simulink model "PartA_19EE10039"  (R2021a)
settings: Solver=FixedStepAuto  StartTime=0.0  StopTime=0.08  FixedStep=1e-7  MaxStep=1e-7  RelTol=1e-6
libraries: simulink x6, spsMonostableLib x6, spsVoltageMeasurementLib x3, spsThreePhaseSourceLib x1, spsThreePhaseTransformerTwoWindingsLib x1, spspowerguiLib x1
settings Model: Creator=Triptendu  LastModifiedBy=mansi
settings SolverCC: AlgebraicLoopSolver=TrustRegion
settings DataIOCC: ReturnWorkspaceOutputs=off
settings DebuggingCC: SFMachineParentedDataDiag=warning

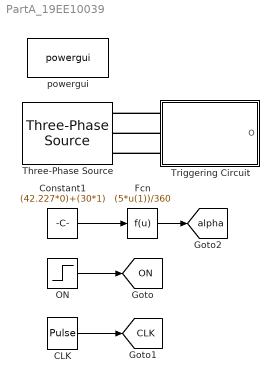
== system PartA_19EE10039 ==
  CLK : DiscretePulseGenerator  PulseType=Time based  Period=40e-6  PulseWidth=50
  Constant1 : Constant  Value=(42.227*0)+(30*1)
  Fcn : Fcn  Expr=(5*u(1))/360
  ON : Step  Time=0.02  SampleTime=0
  Three-Phase Source : spsThreePhaseSourceLib/Three-Phase Source  InternalConnection=Y  VoltagePhases=off  Voltage=220  PhaseAngle=0  Voltage_phases=[25e3 25e3 25e3]/sqrt(3)  PhaseAngles_phases=[0 -120 +120]  Frequency=50  NonIdealSource=on  SpecifyImpedance=off  Resistance=0  Inductance=0  ShortCircuitLevel=100e6  BaseVoltage=220  XRratio=7  BusType=swing  Pref=10e3  Qref=0  Prefabc=[10e3, 10e3, 10e3]  Qrefabc=[0, 0, 0]  Qmin=-inf  Qmax=inf
  Triggering Circuit : Subsystem
  powergui : spspowerguiLib/powergui  Priority=1  SimulationMode=Discrete  SampleTime=1e-8  frequency=60  Iterations=50  frequencyindice=50  Pbase=100e6  ErrMax=1e-4  UnitsV=kV  UnitsW=MW  buscounter=0  FunctionMessages=off  echomessages=off  EnableUseOfTLC=off  CurrentSourceSwitches=off  DisableSnubberDevices=off  DisableRonSwitches=off  DisableVfSwitches=off  DisplayEquations=off  AutomaticDiscreteSolvers=off  SolverType=Backward Euler  Interpol=off  ExternalGateDelay=off  methode=off  Ts=100  x0status=blocks  SPID=on  SwTol=0  HookPort=off  NonlinearTolerance=1e-4  nMaxIteration=100  ContinueOnMaxIteration=off  RestoreLinks=warning  ResistiveCurrentMeasurement=off  Frange=[0:2:500]  Ylog=off  Xlog=on  ShowGrid=off  save=off  variable=ZData  structure=i_ABC_semi  ZoomFFT=on  StartTime=0.04  cycles=2  DisplayStyle=2  fundamental=50  FreqAxis=off  MaxFrequency=1000  frequencyindicesteady=1  RmsSteady=1  display=off
  tag scope: CLK=global, ON=global, alpha=global
  wires:
  ON/1 -> [ON]
  CLK/1 -> [CLK]
  Constant1/1 -> Fcn/1
  Fcn/1 -> [alpha]
  connections:
  Triggering Circuit/LConn1 -- Three-Phase Source/RConn1
  Triggering Circuit/LConn2 -- Three-Phase Source/RConn2
  Triggering Circuit/LConn3 -- Three-Phase Source/RConn3

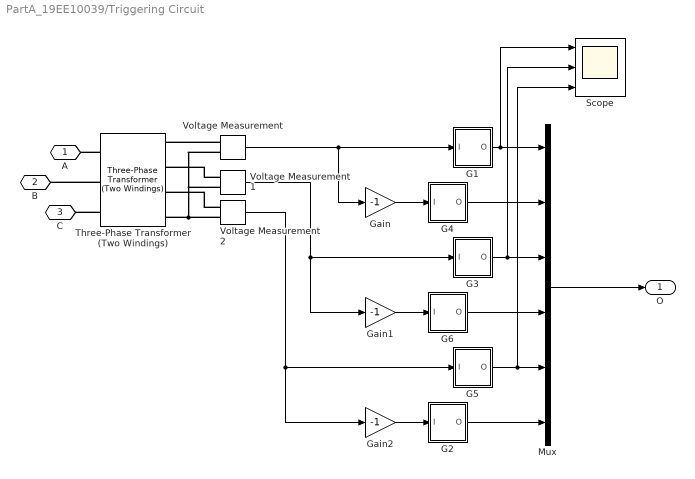
== system PartA_19EE10039/Triggering Circuit ==
  G1 : Subsystem
  G2 : Subsystem
  G3 : Subsystem
  G4 : Subsystem
  G5 : Subsystem
  G6 : Subsystem
  Gain : Gain  Gain=-1
  Gain1 : Gain  Gain=-1
  Gain2 : Gain  Gain=-1
  Mux : Mux  Inputs=6
  Scope : Scope  NumInputPorts=3
  Three-Phase Transformer (Two Windings) : spsThreePhaseTransformerTwoWindingsLib/Three-Phase Transformer (Two Windings)  Winding1Connection=Y  Winding2Connection=Yn  CoreType=Three single-phase transformers  SetSaturation=off  Hysteresis=off  DataFile='hysteresis'  SetInitialFlux=off  Measurements=None  UNITS=SI  NominalPower=[ 100 , 50 ]  Winding1=[220*sqrt(2) 0 0]  Winding2=[5*sqrt(3) 0 0]  Rm=1e6  Lm=1e6  L0=0.5  Saturation=[0 0;0.00044536 1.3723;0.18557 1.7382]  InitialFluxes=[ 0.8 , -0.8 , 0.7 ]  BreakLoop=off  DiscreteSolver=Trapezoidal iterative  DataType=on  TransfoNumber=1
  Voltage Measurement : spsVoltageMeasurementLib/Voltage Measurement  PhasorSimulation=off  OutputType=Complex  PSBequivalent=0
  Voltage Measurement1 : spsVoltageMeasurementLib/Voltage Measurement  PhasorSimulation=off  OutputType=Complex  PSBequivalent=0
  Voltage Measurement2 : spsVoltageMeasurementLib/Voltage Measurement  PhasorSimulation=off  OutputType=Complex  PSBequivalent=0
  A : PMIOPort  Side=Left
  B : PMIOPort  Port=2  Side=Left
  C : PMIOPort  Port=3  Side=Left
  O : Outport
  wires:
  G1/1(O) -> Mux/1, Scope/1
  Gain/1 -> G4/1(I)
  Gain1/1 -> G6/1(I)
  G5/1(O) -> Scope/3, Mux/5
  Voltage Measurement1/1 -> G3/1(I), Gain1/1
  Voltage Measurement2/1 -> G5/1(I), Gain2/1
  Gain2/1 -> G2/1(I)
  Voltage Measurement/1 -> G1/1(I), Gain/1
  G3/1(O) -> Scope/2, Mux/3
  G4/1(O) -> Mux/2
  G2/1(O) -> Mux/6
  G6/1(O) -> Mux/4
  Mux/1 -> O/1
  connections:
  Voltage Measurement2/LConn2 -- Voltage Measurement/LConn2 -- Voltage Measurement1/LConn2 -- Three-Phase Transformer (Two Windings)/RConn4
  Voltage Measurement2/LConn1 -- Three-Phase Transformer (Two Windings)/RConn3
  Voltage Measurement/LConn1 -- Three-Phase Transformer (Two Windings)/RConn1
  Three-Phase Transformer (Two Windings)/LConn2 -- B/RConn1
  Voltage Measurement1/LConn1 -- Three-Phase Transformer (Two Windings)/RConn2
  Three-Phase Transformer (Two Windings)/LConn1 -- A/RConn1
  Three-Phase Transformer (Two Windings)/LConn3 -- C/RConn1

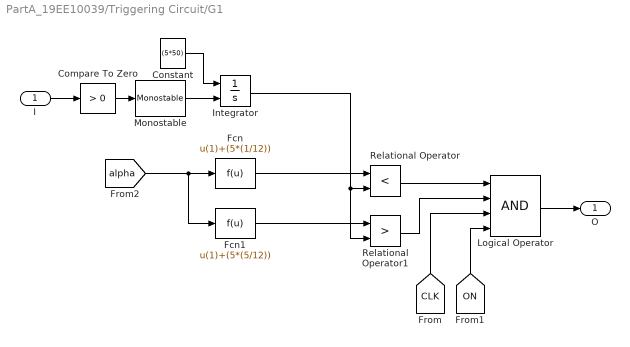
== system PartA_19EE10039/Triggering Circuit/G1 ==
  I : Inport
  Compare To Zero : simulink/Logic and Bit Operations/Compare To Zero  relop=>  OutDataTypeStr=boolean
  Constant : Constant  Value=(5*50)
  Fcn : Fcn  Expr=u(1)+(5*(1/12))
  Fcn1 : Fcn  Expr=u(1)+(5*(5/12))
  Integrator : Integrator  ExternalReset=rising
  Logical Operator : Logic  Inputs=4  AllPortsSameDT=off  OutDataTypeStr=boolean
  Monostable : spsMonostableLib/Monostable  EdgeDetect=Rising  PulseDuration=10e-6  ic=0  Ts=1e-6
      settings: SourceProductBaseCode=PS
  Relational Operator : RelationalOperator  Operator=<  OutDataTypeStr=boolean  RndMeth=Simplest
  Relational Operator1 : RelationalOperator  Operator=>  OutDataTypeStr=boolean  RndMeth=Simplest
  O : Outport
  wires:
  [CLK] -> Logical Operator/3
  Relational Operator1/1 -> Logical Operator/2
  Compare To Zero/1 -> Monostable/1
  Relational Operator/1 -> Logical Operator/1
  [alpha] -> Fcn1/1, Fcn/1
  [ON] -> Logical Operator/4
  Fcn1/1 -> Relational Operator1/1
  Fcn/1 -> Relational Operator/1
  Constant/1 -> Integrator/1
  Monostable/1 -> Integrator/2
  I/1 -> Compare To Zero/1
  Logical Operator/1 -> O/1
  Integrator/1 -> Relational Operator1/2, Relational Operator/2

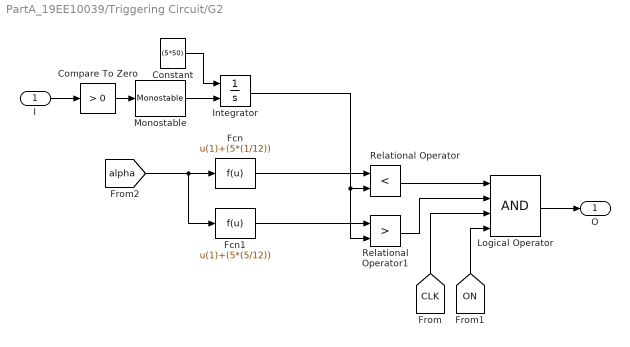
== system PartA_19EE10039/Triggering Circuit/G2 ==
  I : Inport
  Compare To Zero : simulink/Logic and Bit Operations/Compare To Zero  relop=>  OutDataTypeStr=boolean
  Constant : Constant  Value=(5*50)
  Fcn : Fcn  Expr=u(1)+(5*(1/12))
  Fcn1 : Fcn  Expr=u(1)+(5*(5/12))
  Integrator : Integrator  ExternalReset=rising
  Logical Operator : Logic  Inputs=4  AllPortsSameDT=off  OutDataTypeStr=boolean
  Monostable : spsMonostableLib/Monostable  EdgeDetect=Rising  PulseDuration=10e-6  ic=0  Ts=1e-6
      settings: SourceProductBaseCode=PS
  Relational Operator : RelationalOperator  Operator=<  OutDataTypeStr=boolean  RndMeth=Simplest
  Relational Operator1 : RelationalOperator  Operator=>  OutDataTypeStr=boolean  RndMeth=Simplest
  O : Outport
  wires:
  Integrator/1 -> Relational Operator/2, Relational Operator1/2
  Logical Operator/1 -> O/1
  I/1 -> Compare To Zero/1
  Monostable/1 -> Integrator/2
  Constant/1 -> Integrator/1
  Fcn/1 -> Relational Operator/1
  Fcn1/1 -> Relational Operator1/1
  [ON] -> Logical Operator/4
  [alpha] -> Fcn/1, Fcn1/1
  Relational Operator/1 -> Logical Operator/1
  Compare To Zero/1 -> Monostable/1
  Relational Operator1/1 -> Logical Operator/2
  [CLK] -> Logical Operator/3

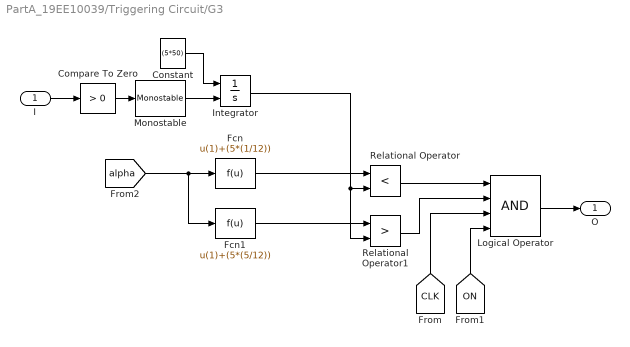
== system PartA_19EE10039/Triggering Circuit/G3 ==
  I : Inport
  Compare To Zero : simulink/Logic and Bit Operations/Compare To Zero  relop=>  OutDataTypeStr=boolean
  Constant : Constant  Value=(5*50)
  Fcn : Fcn  Expr=u(1)+(5*(1/12))
  Fcn1 : Fcn  Expr=u(1)+(5*(5/12))
  Integrator : Integrator  ExternalReset=rising
  Logical Operator : Logic  Inputs=4  AllPortsSameDT=off  OutDataTypeStr=boolean
  Monostable : spsMonostableLib/Monostable  EdgeDetect=Rising  PulseDuration=10e-6  ic=0  Ts=1e-6
      settings: SourceProductBaseCode=PS
  Relational Operator : RelationalOperator  Operator=<  OutDataTypeStr=boolean  RndMeth=Simplest
  Relational Operator1 : RelationalOperator  Operator=>  OutDataTypeStr=boolean  RndMeth=Simplest
  O : Outport
  wires:
  [CLK] -> Logical Operator/3
  Relational Operator1/1 -> Logical Operator/2
  Compare To Zero/1 -> Monostable/1
  Relational Operator/1 -> Logical Operator/1
  [alpha] -> Fcn1/1, Fcn/1
  [ON] -> Logical Operator/4
  Fcn1/1 -> Relational Operator1/1
  Fcn/1 -> Relational Operator/1
  Constant/1 -> Integrator/1
  Monostable/1 -> Integrator/2
  I/1 -> Compare To Zero/1
  Logical Operator/1 -> O/1
  Integrator/1 -> Relational Operator1/2, Relational Operator/2

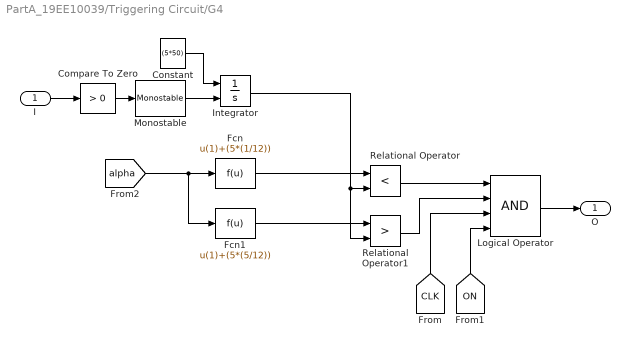
== system PartA_19EE10039/Triggering Circuit/G4 ==
  I : Inport
  Compare To Zero : simulink/Logic and Bit Operations/Compare To Zero  relop=>  OutDataTypeStr=boolean
  Constant : Constant  Value=(5*50)
  Fcn : Fcn  Expr=u(1)+(5*(1/12))
  Fcn1 : Fcn  Expr=u(1)+(5*(5/12))
  Integrator : Integrator  ExternalReset=rising
  Logical Operator : Logic  Inputs=4  AllPortsSameDT=off  OutDataTypeStr=boolean
  Monostable : spsMonostableLib/Monostable  EdgeDetect=Rising  PulseDuration=10e-6  ic=0  Ts=1e-6
      settings: SourceProductBaseCode=PS
  Relational Operator : RelationalOperator  Operator=<  OutDataTypeStr=boolean  RndMeth=Simplest
  Relational Operator1 : RelationalOperator  Operator=>  OutDataTypeStr=boolean  RndMeth=Simplest
  O : Outport
  wires:
  Integrator/1 -> Relational Operator/2, Relational Operator1/2
  Logical Operator/1 -> O/1
  I/1 -> Compare To Zero/1
  Monostable/1 -> Integrator/2
  Constant/1 -> Integrator/1
  Fcn/1 -> Relational Operator/1
  Fcn1/1 -> Relational Operator1/1
  [ON] -> Logical Operator/4
  [alpha] -> Fcn/1, Fcn1/1
  Relational Operator/1 -> Logical Operator/1
  Compare To Zero/1 -> Monostable/1
  Relational Operator1/1 -> Logical Operator/2
  [CLK] -> Logical Operator/3

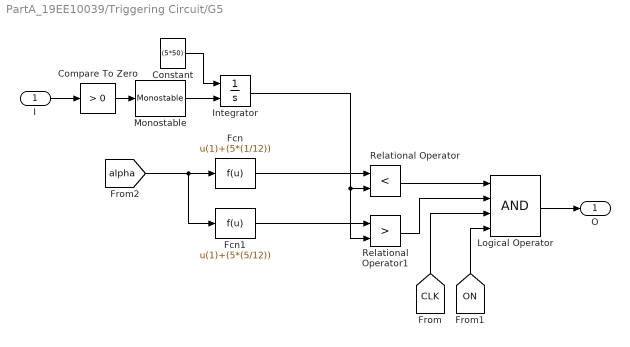
== system PartA_19EE10039/Triggering Circuit/G5 ==
  I : Inport
  Compare To Zero : simulink/Logic and Bit Operations/Compare To Zero  relop=>  OutDataTypeStr=boolean
  Constant : Constant  Value=(5*50)
  Fcn : Fcn  Expr=u(1)+(5*(1/12))
  Fcn1 : Fcn  Expr=u(1)+(5*(5/12))
  Integrator : Integrator  ExternalReset=rising
  Logical Operator : Logic  Inputs=4  AllPortsSameDT=off  OutDataTypeStr=boolean
  Monostable : spsMonostableLib/Monostable  EdgeDetect=Rising  PulseDuration=10e-6  ic=0  Ts=1e-6
      settings: SourceProductBaseCode=PS
  Relational Operator : RelationalOperator  Operator=<  OutDataTypeStr=boolean  RndMeth=Simplest
  Relational Operator1 : RelationalOperator  Operator=>  OutDataTypeStr=boolean  RndMeth=Simplest
  O : Outport
  wires:
  [CLK] -> Logical Operator/3
  Relational Operator1/1 -> Logical Operator/2
  Compare To Zero/1 -> Monostable/1
  Relational Operator/1 -> Logical Operator/1
  [alpha] -> Fcn1/1, Fcn/1
  [ON] -> Logical Operator/4
  Fcn1/1 -> Relational Operator1/1
  Fcn/1 -> Relational Operator/1
  Constant/1 -> Integrator/1
  Monostable/1 -> Integrator/2
  I/1 -> Compare To Zero/1
  Logical Operator/1 -> O/1
  Integrator/1 -> Relational Operator1/2, Relational Operator/2

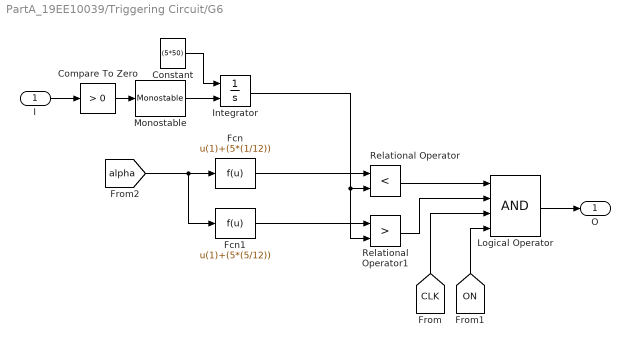
== system PartA_19EE10039/Triggering Circuit/G6 ==
  I : Inport
  Compare To Zero : simulink/Logic and Bit Operations/Compare To Zero  relop=>  OutDataTypeStr=boolean
  Constant : Constant  Value=(5*50)
  Fcn : Fcn  Expr=u(1)+(5*(1/12))
  Fcn1 : Fcn  Expr=u(1)+(5*(5/12))
  Integrator : Integrator  ExternalReset=rising
  Logical Operator : Logic  Inputs=4  AllPortsSameDT=off  OutDataTypeStr=boolean
  Monostable : spsMonostableLib/Monostable  EdgeDetect=Rising  PulseDuration=10e-6  ic=0  Ts=1e-6
      settings: SourceProductBaseCode=PS
  Relational Operator : RelationalOperator  Operator=<  OutDataTypeStr=boolean  RndMeth=Simplest
  Relational Operator1 : RelationalOperator  Operator=>  OutDataTypeStr=boolean  RndMeth=Simplest
  O : Outport
  wires:
  Integrator/1 -> Relational Operator/2, Relational Operator1/2
  Logical Operator/1 -> O/1
  I/1 -> Compare To Zero/1
  Monostable/1 -> Integrator/2
  Constant/1 -> Integrator/1
  Fcn/1 -> Relational Operator/1
  Fcn1/1 -> Relational Operator1/1
  [ON] -> Logical Operator/4
  [alpha] -> Fcn/1, Fcn1/1
  Relational Operator/1 -> Logical Operator/1
  Compare To Zero/1 -> Monostable/1
  Relational Operator1/1 -> Logical Operator/2
  [CLK] -> Logical Operator/3
